simulink model "ex1_1"  (R2021b)
settings: Solver=VariableStepAuto  StartTime=0.0  StopTime=10.0  RelTol=1e-3
settings Model: Creator=86137  LastModifiedBy=86137

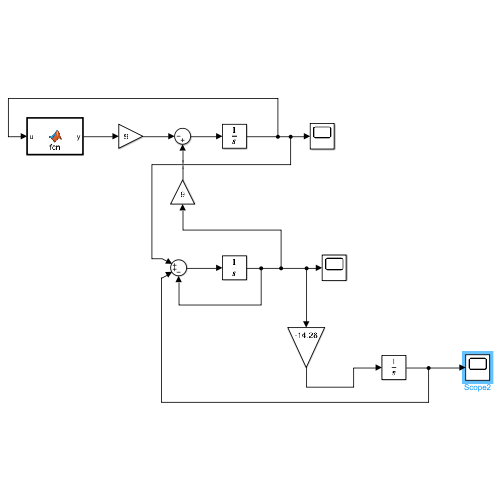
[thumbnail: Simulink's stored preview of the top-level diagram]
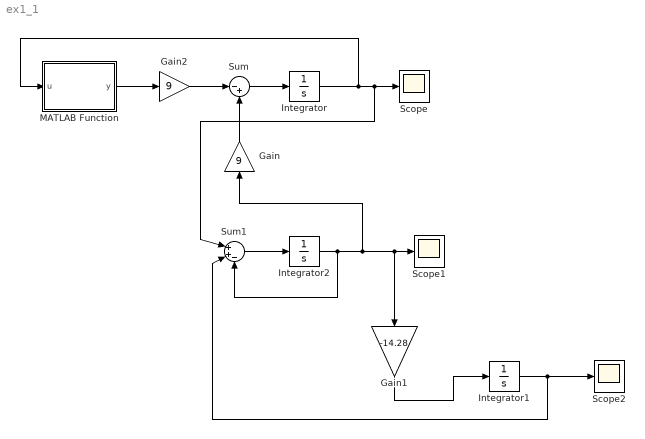
== system ex1_1 ==
  Gain : Gain  Gain=9
  Gain1 : Gain  Gain=-14.28
  Gain2 : Gain  Gain=9
  Integrator : Integrator  InitialCondition=1
  Integrator1 : Integrator  InitialCondition=3
  Integrator2 : Integrator  InitialCondition=2
  MATLAB Function : MATLAB Function  TreatAsAtomicUnit=on
  Scope : Scope
  Scope1 : Scope
  Scope2 : Scope
  Sum : Sum  Inputs=|-+
  Sum1 : Sum  Inputs=|++-
  wires:
  Gain2/1 -> Sum/1
  MATLAB Function/1(y) -> Gain2/1
  Sum1/1 -> Integrator2/1
  Integrator1/1 -> Sum1/2, Scope2/1
  Integrator2/1 -> Sum1/3, Scope1/1, Gain1/1, Gain/1
  Sum/1 -> Integrator/1
  Gain1/1 -> Integrator1/1
  Integrator/1 -> MATLAB Function/1(u), Sum1/1, Scope/1
  Gain/1 -> Sum/2

== matlab function ex1_1/MATLAB Function ==
  data: u input; y output
function y = fcn(u)

y =(2/7)* u+(1/2)*(-3/7)*(abs(u+1)-abs(u-1));
